simulink model "Standalone_Speed_MPC"  (R2025b)
settings: Solver=FixedStepDiscrete  StartTime=0.0  StopTime=20  FixedStep=1e-4  MaxStep=1e-4  RelTol=1e-3
settings Model: SimulationMode=processor-in-the-loop (pil)  Creator=Harish  LastModifiedBy=Harish
settings DataIOCC: ExternalInput=in_w_ref, in_omega_m, in_Vdc, in_Rs, in_Ld, in_Lq, in_PsiPM, in_control_mode, in_J_est, in_B_est  LoadExternalInput=on  OutputSaveName=yout_sil
settings OptimizationCC: DefaultParameterBehavior=Inlined  EnhancedBackFolding=on  PassReuseOutputArgsAs=Individual arguments  ZeroExternalMemoryAtStartup=off  ZeroInternalMemoryAtStartup=off  OptimizeBlockOrder=speed  DifferentSizesBufferReuse=on  OptimizationCustomize=off  EfficientTunableParamExpr=on
settings DebuggingCC: ParameterTunabilityLossMsg=error
settings HardwareCC: TargetLargestAtomicInteger=Long  TargetLargestAtomicFloat=Double  TargetIntDivRoundTo=Zero  TargetEndianess=LittleEndian  TargetHWDeviceType=ARM Compatible->ARM Cortex-M
settings SFSimCC: MATLABDynamicMemAlloc=off
settings RTWCC: SystemTargetFile=ert.tlc  TemplateMakefile=ert_default_tmf  GenerateReport=on  Toolchain=MinGW64 | gmake (64-bit Windows)  GenerateCodeMetricsReport=on  Description=Embedded Coder
settings CodeAppCC: ForceParamTrailComments=on  IgnoreCustomStorageClasses=off  OperatorAnnotations=on  SimulinkDataObjDesc=on  SFDataObjDesc=on  InsertBlockDesc=on
settings ERTTargetCC: ERTCustomFileTemplate=example_file_process.tlc  TargetLangStandard=C99 (ISO)  GenerateSampleERTMain=on  SupportContinuousTime=on

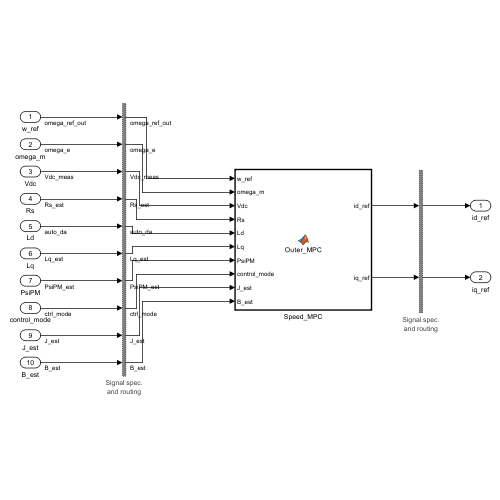
[thumbnail: Simulink's stored preview of the top-level diagram]
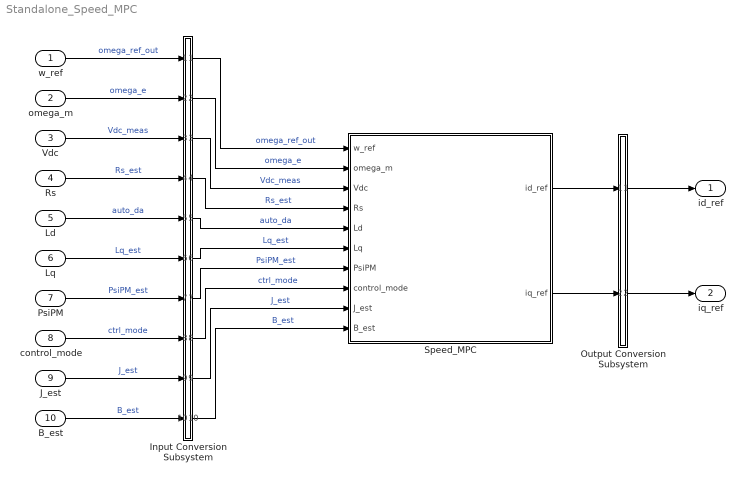
== system Standalone_Speed_MPC ==
  w_ref : Inport  OutDataTypeStr=double  PortDimensions=[1]  SampleTime=0.0001
  omega_m : Inport  Port=2  OutDataTypeStr=double  PortDimensions=[1]  SampleTime=0.0001
  Vdc : Inport  Port=3  OutDataTypeStr=double  PortDimensions=[1]  SampleTime=0.0001
  Rs : Inport  Port=4  OutDataTypeStr=double  PortDimensions=[1]  SampleTime=0.0001
  Ld : Inport  Port=5  OutDataTypeStr=double  PortDimensions=[1]  SampleTime=0.0001
  Lq : Inport  Port=6  OutDataTypeStr=double  PortDimensions=[1]  SampleTime=0.0001
  PsiPM : Inport  Port=7  OutDataTypeStr=double  PortDimensions=[1]  SampleTime=0.0001
  control_mode : Inport  Port=8  OutDataTypeStr=double  PortDimensions=[1]  SampleTime=0.0001
  J_est : Inport  Port=9  OutDataTypeStr=double  PortDimensions=[1]  SampleTime=0.0001
  B_est : Inport  Port=10  OutDataTypeStr=double  PortDimensions=[1]  SampleTime=0.0001
  Input Conversion Subsystem : Subsystem  Tag=__SLT_ICS__  Description=|
      | Signal spec.
      | and routing
      settings: AttributesFormatString=%<Description>
  Output Conversion Subsystem : Subsystem  Tag=__SLT_OCS__  Description=|
      | Signal spec.
      | and routing
      settings: AttributesFormatString=%<Description>
  Speed_MPC : MATLAB Function  TreatAsAtomicUnit=on
  id_ref : Outport
  iq_ref : Outport  Port=2
  wires:
  w_ref/1 -> Input Conversion Subsystem/1(Inport_1)  "omega_ref_out"
  omega_m/1 -> Input Conversion Subsystem/2(Inport_2)  "omega_e"
  Vdc/1 -> Input Conversion Subsystem/3(Inport_3)  "Vdc_meas"
  Rs/1 -> Input Conversion Subsystem/4(Inport_4)  "Rs_est"
  Ld/1 -> Input Conversion Subsystem/5(Inport_5)  "auto_da"
  Lq/1 -> Input Conversion Subsystem/6(Inport_6)  "Lq_est"
  PsiPM/1 -> Input Conversion Subsystem/7(Inport_7)  "PsiPM_est"
  control_mode/1 -> Input Conversion Subsystem/8(Inport_8)  "ctrl_mode"
  J_est/1 -> Input Conversion Subsystem/9(Inport_9)  "J_est"
  B_est/1 -> Input Conversion Subsystem/10(Inport_10)  "B_est"
  Output Conversion Subsystem/1(Outport_1) -> id_ref/1
  Output Conversion Subsystem/2(Outport_2) -> iq_ref/1
  Input Conversion Subsystem/1(Outport_1) -> Speed_MPC/1(w_ref)  "omega_ref_out"
  Input Conversion Subsystem/2(Outport_2) -> Speed_MPC/2(omega_m)  "omega_e"
  Input Conversion Subsystem/3(Outport_3) -> Speed_MPC/3(Vdc)  "Vdc_meas"
  Input Conversion Subsystem/4(Outport_4) -> Speed_MPC/4(Rs)  "Rs_est"
  Input Conversion Subsystem/5(Outport_5) -> Speed_MPC/5(Ld)  "auto_da"
  Input Conversion Subsystem/6(Outport_6) -> Speed_MPC/6(Lq)  "Lq_est"
  Input Conversion Subsystem/7(Outport_7) -> Speed_MPC/7(PsiPM)  "PsiPM_est"
  Input Conversion Subsystem/8(Outport_8) -> Speed_MPC/8(control_mode)  "ctrl_mode"
  Input Conversion Subsystem/9(Outport_9) -> Speed_MPC/9(J_est)  "J_est"
  Input Conversion Subsystem/10(Outport_10) -> Speed_MPC/10(B_est)  "B_est"
  Speed_MPC/1(id_ref) -> Output Conversion Subsystem/1(Inport_1)
  Speed_MPC/2(iq_ref) -> Output Conversion Subsystem/2(Inport_2)

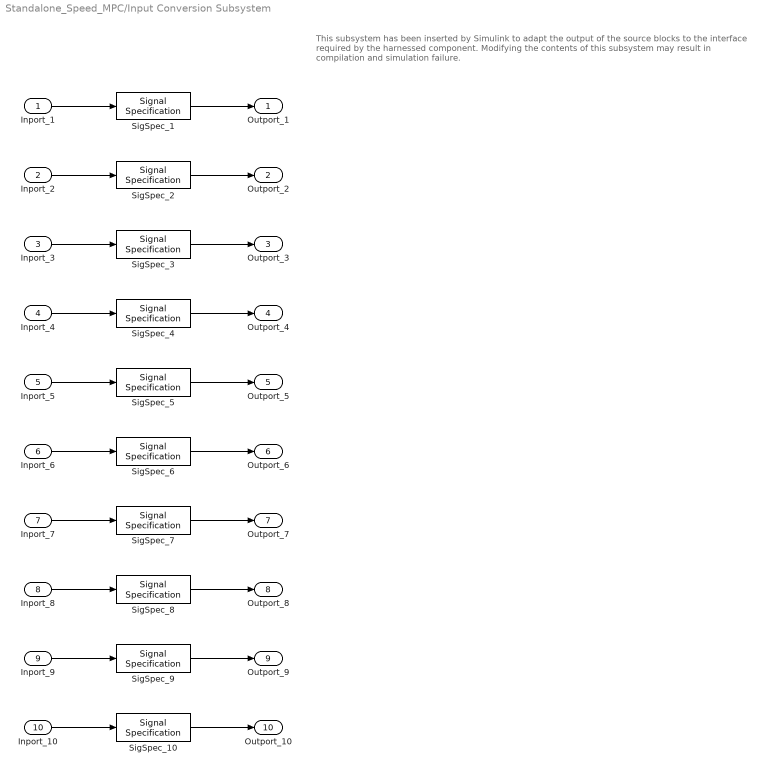
== system Standalone_Speed_MPC/Input Conversion Subsystem ==
  note: This subsystem has been inserted by Simulink to adapt the output of the source blocks to the interface required by the harnessed component.
      |  Modifying the contents of this subsystem may result in compilation and simulation failure.
  Inport_1 : Inport
  Inport_2 : Inport  Port=2
  Inport_3 : Inport  Port=3
  Inport_4 : Inport  Port=4
  Inport_5 : Inport  Port=5
  Inport_6 : Inport  Port=6
  Inport_7 : Inport  Port=7
  Inport_8 : Inport  Port=8
  Inport_9 : Inport  Port=9
  Inport_10 : Inport  Port=10
  SigSpec_{1..10} (10 alike) : SignalSpecification  OutDataTypeStr=double  Dimensions=[1]
  Outport_1 : Outport
  Outport_2 : Outport  Port=2
  Outport_3 : Outport  Port=3
  Outport_4 : Outport  Port=4
  Outport_5 : Outport  Port=5
  Outport_6 : Outport  Port=6
  Outport_7 : Outport  Port=7
  Outport_8 : Outport  Port=8
  Outport_9 : Outport  Port=9
  Outport_10 : Outport  Port=10
  wires:
  SigSpec_1/1 -> Outport_1/1
  Inport_1/1 -> SigSpec_1/1
  SigSpec_2/1 -> Outport_2/1
  Inport_2/1 -> SigSpec_2/1
  SigSpec_3/1 -> Outport_3/1
  Inport_3/1 -> SigSpec_3/1
  SigSpec_4/1 -> Outport_4/1
  Inport_4/1 -> SigSpec_4/1
  SigSpec_5/1 -> Outport_5/1
  Inport_5/1 -> SigSpec_5/1
  SigSpec_6/1 -> Outport_6/1
  Inport_6/1 -> SigSpec_6/1
  SigSpec_7/1 -> Outport_7/1
  Inport_7/1 -> SigSpec_7/1
  SigSpec_8/1 -> Outport_8/1
  Inport_8/1 -> SigSpec_8/1
  SigSpec_9/1 -> Outport_9/1
  Inport_9/1 -> SigSpec_9/1
  SigSpec_10/1 -> Outport_10/1
  Inport_10/1 -> SigSpec_10/1

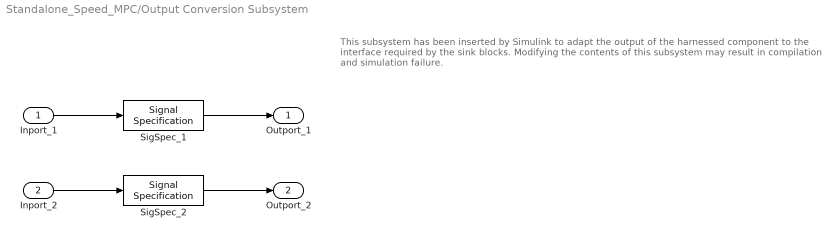
== system Standalone_Speed_MPC/Output Conversion Subsystem ==
  note: This subsystem has been inserted by Simulink to adapt the output of the harnessed component to the interface required by the sink blocks.
      |  Modifying the contents of this subsystem may result in compilation and simulation failure.
  Inport_1 : Inport
  Inport_2 : Inport  Port=2
  SigSpec_1 : SignalSpecification  OutDataTypeStr=double  Dimensions=[1]
  SigSpec_2 : SignalSpecification  OutDataTypeStr=double  Dimensions=[1]
  Outport_1 : Outport
  Outport_2 : Outport  Port=2
  wires:
  Inport_1/1 -> SigSpec_1/1
  SigSpec_1/1 -> Outport_1/1
  Inport_2/1 -> SigSpec_2/1
  SigSpec_2/1 -> Outport_2/1

== matlab function Standalone_Speed_MPC/Speed_MPC ==
  data: w_ref input double size=1; id_ref output double size=1; omega_m input double size=1; Vdc input double size=1; Rs input double size=1; Ld input double size=1; Lq input double size=1; PsiPM input double size=1; iq_ref output double size=1; control_mode input; J_est input; B_est input
function [id_ref, iq_ref] = Outer_MPC(w_ref, omega_m, Vdc, Rs, Ld, Lq, PsiPM, control_mode, J_est, B_est)
    % Cascaded Multi-Rate Speed MPC & Analytical Smooth MTPA/FW Optimizer
    % control_mode: 1 = Active Speed Control, 0/2 = Disabled / Tuning Mode
    
    id_ref = zeros(1, 1, 'double');
    iq_ref = zeros(1, 1, 'double');
    
    pp = 6.0;         % i3 motor pole pairs
    I_max = 565.0;    % Maximum phase current (A peak)
    Ts_dt = 1e-4;     % Discrete sample interval (100 us / 10 kHz)
    
    persistent omega_filt;
    persistent e_int;
    
    if isempty(omega_filt)
        omega_filt = double(omega_m);
        e_int = 0.0;
    end
    
    % Control Mode Bypass during AutoTuning (mode ~= 1)
    if control_mode ~= 1
        omega_filt = double(omega_m);
        e_int = 0.0;
        id_ref(1) = 0.0;
        iq_ref(1) = 0.0;
        return;
    end
    
    % Parameter extraction and protective lower bounds
    J_val = max(double(J_est), 0.001);
    B_val = max(double(B_est), 0.0);
    Psi_val = max(double(PsiPM), 0.005);
    Ld_val = max(double(Ld), 1e-6);
    Lq_val = max(double(Lq), 1e-6);
    dL = Lq_val - Ld_val;
    
    % 1. Low-pass filter raw measured speed to eliminate PWM carrier derivative chatter
    alpha_w = 0.95;
    omega_filt = alpha_w * omega_filt + (1.0 - alpha_w) * double(omega_m);
    
    % Convert to mechanical speed
    w_ref_mech = double(w_ref) / pp;
    w_mech = omega_filt / pp;
    
    % 2. Speed MPC control law (Matched to inertia J)
    e_w = w_ref_mech - w_mech;
    e_int = e_int + e_w * Ts_dt;
    
    Kp_w = 6.5 * (J_val / 0.0867);
    Ki_w = 120.0 * (J_val / 0.0867);
    
    Te_cmd = Kp_w * e_w + Ki_w * e_int + B_val * w_mech;
    
    % Anti-windup clamping
    if Te_cmd > 258.2
        Te_cmd = 258.2;
        e_int = e_int - e_w * Ts_dt;
    elseif Te_cmd < -258.2
        Te_cmd = -258.2;
        e_int = e_int - e_w * Ts_dt;
    end
    
    % 3. Analytical Smooth MTPA Trajectory
    if abs(Te_cmd) < 1e-3 || dL < 1e-7
        id_mtpa = 0.0;
        iq_mtpa = Te_cmd / (1.5 * pp * Psi_val);
    else
        iq_lin = Te_cmd / (1.5 * pp * Psi_val);
        id_mtpa = - (dL / (2.0 * Psi_val)) * (iq_lin^2);
        if id_mtpa < -0.45 * I_max
            id_mtpa = -0.45 * I_max;
        end
        
        denom = Psi_val + (Ld_val - Lq_val) * id_mtpa;
        if abs(denom) < 1e-4
            denom = 1e-4;
        end
        iq_mtpa = Te_cmd / (1.5 * pp * denom);
    end
    
    % 4. Analytical Closed-Form Voltage Ellipse Field Weakening
    V_max = (double(Vdc) / sqrt(3.0)) * 0.95;
    omega_e = max(abs(double(omega_m)), 1.0);
    
    Vd_est = -omega_e * Lq_val * iq_mtpa;
    Vq_est = omega_e * Ld_val * id_mtpa + omega_e * Psi_val;
    V_est = sqrt(Vd_est^2 + Vq_est^2);
    
    if V_est > V_max && omega_e > 2000.0
        V_lim = V_max / omega_e;
        max_iq_sq = max(0.0, (V_lim^2) / (Lq_val^2));
        if (iq_mtpa^2) > 0.90 * max_iq_sq
            iq_fw = sign(iq_mtpa) * sqrt(0.90 * max_iq_sq);
        else
            iq_fw = iq_mtpa;
        end
        
        val_under_sqrt = max(0.0, V_lim^2 - (Lq_val * iq_fw)^2);
        id_fw = (-Psi_val + sqrt(val_under_sqrt)) / Ld_val;
        if id_fw > id_mtpa
            id_fw = (-Psi_val - sqrt(val_under_sqrt)) / Ld_val;
        end
        id_out = id_fw;
        iq_out = iq_fw;
    else
        id_out = id_mtpa;
        iq_out = iq_mtpa;
    end
    
    % 5. Stator Current Circle Clamp
    I_tot = sqrt(id_out^2 + iq_out^2);
    if I_tot > I_max
        id_out = id_out * (I_max / I_tot);
        iq_out = iq_out * (I_max / I_tot);
    end
    
    id_ref(1) = id_out;
    iq_ref(1) = iq_out;
end
